simulink library "ESTS_UOD"  (R2024b)
settings: Solver=VariableStepAuto  StartTime=0.0  StopTime=10.0  RelTol=1e-3
libraries: ESTS_UOD_YawRateDeadZone x1, ESTS_UOD_CornrgDir x1, ESTS_UOD_YawRateDifLatRef x1, ESTS_UOD_AgrVSideSlipReDifLatRef x1, ESTS_UOD_FacUnderSteer x1, ESTS_UOD_FacOverSteer x1, VUT_lib x1
settings Model: Creator=blatak  LastModifiedBy=blatak
settings ModelReferenceCC: EnableRefExpFcnMdlSchedulingChecks=on
settings RTWCC: GPUComputeCapability=3.5

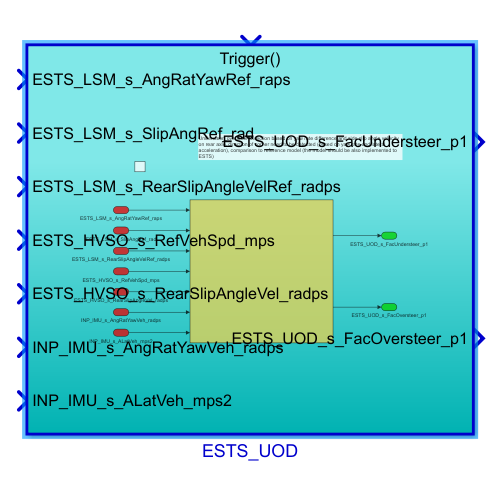
[thumbnail: Simulink's stored preview of the top-level diagram]
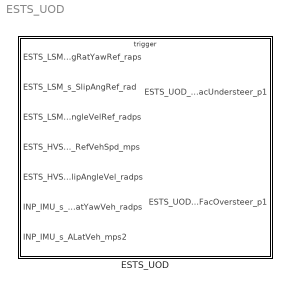
== system ESTS_UOD ==
  ESTS_UOD : Subsystem

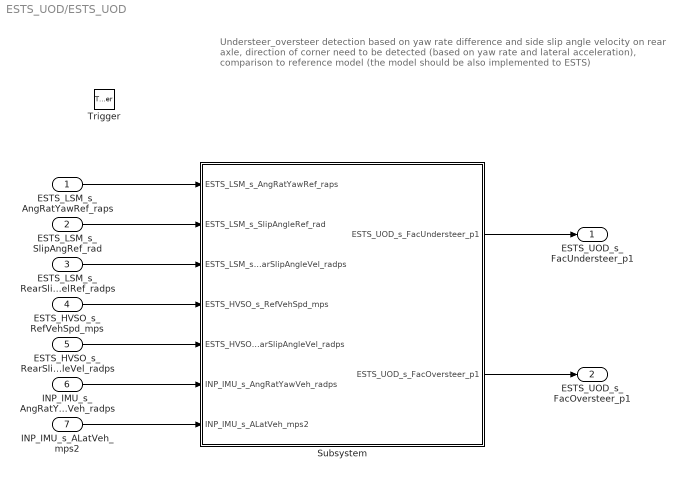
== system ESTS_UOD/ESTS_UOD ==
  note: Understeer_oversteer detection based on yaw rate difference and side slip angle velocity on rear axle, direction of corner need to be detected (based on yaw rate and lateral acceleration), comparison to reference model (the model should be also implemented to ESTS)
  ESTS_LSM_s_AngRatYawRef_raps : Inport
  ESTS_LSM_s_SlipAngRef_rad : Inport  Port=2
  ESTS_LSM_s_RearSlipAngleVelRef_radps : Inport  Port=3
  ESTS_HVSO_s_RefVehSpd_mps : Inport  Port=4
  ESTS_HVSO_s_RearSlipAngleVel_radps : Inport  Port=5
  INP_IMU_s_AngRatYawVeh_radps : Inport  Port=6
  INP_IMU_s_ALatVeh_mps2 : Inport  Port=7
  Trigger : TriggerPort  TriggerType=function-call  VariantControl=(inherit)  PortDimensions=1
  Subsystem : Subsystem
  ESTS_UOD_s_FacUndersteer_p1 : Outport
  ESTS_UOD_s_FacOversteer_p1 : Outport  Port=2
  wires:
  ESTS_LSM_s_RearSlipAngleVelRef_radps/1 -> Subsystem/3(ESTS_LSM_s_RearSlipAngleVel_radps)
  ESTS_HVSO_s_RefVehSpd_mps/1 -> Subsystem/4(ESTS_HVSO_s_RefVehSpd_mps)
  ESTS_HVSO_s_RearSlipAngleVel_radps/1 -> Subsystem/5(ESTS_HVSO_s_RearSlipAngleVel_radps)
  ESTS_LSM_s_SlipAngRef_rad/1 -> Subsystem/2(ESTS_LSM_s_SlipAngleRef_rad)
  ESTS_LSM_s_AngRatYawRef_raps/1 -> Subsystem/1(ESTS_LSM_s_AngRatYawRef_raps)
  Subsystem/2(ESTS_UOD_s_FacOversteer_p1) -> ESTS_UOD_s_FacOversteer_p1/1
  Subsystem/1(ESTS_UOD_s_FacUndersteer_p1) -> ESTS_UOD_s_FacUndersteer_p1/1
  INP_IMU_s_AngRatYawVeh_radps/1 -> Subsystem/6(INP_IMU_s_AngRatYawVeh_radps)
  INP_IMU_s_ALatVeh_mps2/1 -> Subsystem/7(INP_IMU_s_ALatVeh_mps2)

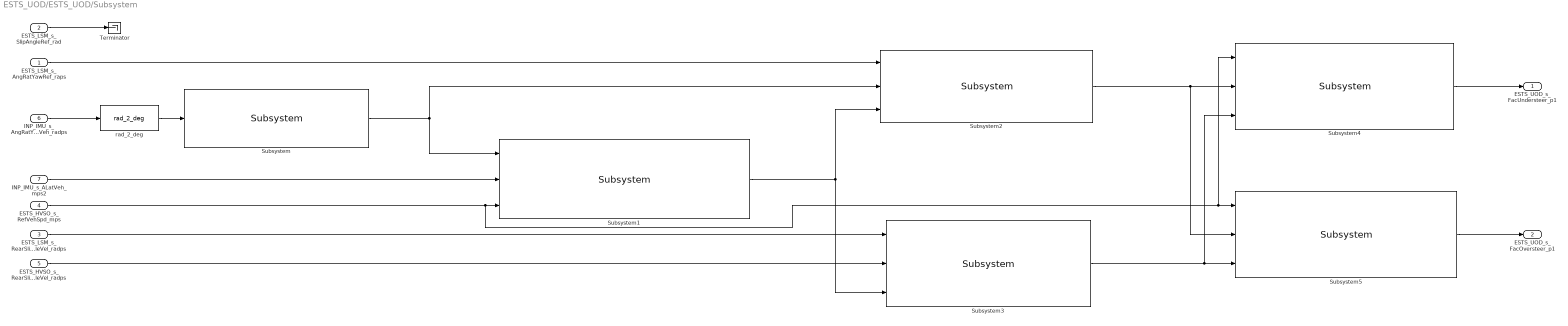
== system ESTS_UOD/ESTS_UOD/Subsystem ==
  ESTS_LSM_s_AngRatYawRef_raps : Inport
  ESTS_LSM_s_SlipAngleRef_rad : Inport  Port=2
  ESTS_LSM_s_RearSlipAngleVel_radps : Inport  Port=3
  ESTS_HVSO_s_RefVehSpd_mps : Inport  Port=4
  ESTS_HVSO_s_RearSlipAngleVel_radps : Inport  Port=5
  INP_IMU_s_AngRatYawVeh_radps : Inport  Port=6
  INP_IMU_s_ALatVeh_mps2 : Inport  Port=7
  Subsystem : ESTS_UOD_YawRateDeadZone/Subsystem  SystemSampleTime=-1  VariantActivationTime=update diagram  AllowFlexibleInterface=on  Latency=0  AutoFrameSizeCalculation=off
  Subsystem1 : ESTS_UOD_CornrgDir/Subsystem  SystemSampleTime=-1  VariantActivationTime=update diagram  AllowFlexibleInterface=on  Latency=0  AutoFrameSizeCalculation=off
  Subsystem2 : ESTS_UOD_YawRateDifLatRef/Subsystem  SystemSampleTime=-1  VariantActivationTime=update diagram  AllowFlexibleInterface=on  Latency=0  AutoFrameSizeCalculation=off
  Subsystem3 : ESTS_UOD_AgrVSideSlipReDifLatRef/Subsystem  SystemSampleTime=-1  VariantActivationTime=update diagram  AllowFlexibleInterface=on  Latency=0  AutoFrameSizeCalculation=off
  Subsystem4 : ESTS_UOD_FacUnderSteer/Subsystem  SystemSampleTime=-1  VariantActivationTime=update diagram  AllowFlexibleInterface=on  Latency=0  AutoFrameSizeCalculation=off
  Subsystem5 : ESTS_UOD_FacOverSteer/Subsystem  SystemSampleTime=-1  VariantActivationTime=update diagram  AllowFlexibleInterface=on  Latency=0  AutoFrameSizeCalculation=off
  Terminator : Terminator
  rad_2_deg : VUT_lib/rad_2_deg  SystemSampleTime=-1  VariantActivationTime=update diagram  AllowFlexibleInterface=on  Latency=0  AutoFrameSizeCalculation=off
  ESTS_UOD_s_FacUndersteer_p1 : Outport
  ESTS_UOD_s_FacOversteer_p1 : Outport  Port=2
  wires:
  INP_IMU_s_AngRatYawVeh_radps/1 -> rad_2_deg/1
  rad_2_deg/1 -> Subsystem/1
  INP_IMU_s_ALatVeh_mps2/1 -> Subsystem1/2
  Subsystem/1 -> Subsystem1/1, Subsystem2/2
  ESTS_LSM_s_RearSlipAngleVel_radps/1 -> Subsystem3/1
  ESTS_LSM_s_SlipAngleRef_rad/1 -> Terminator/1
  ESTS_HVSO_s_RearSlipAngleVel_radps/1 -> Subsystem3/2
  Subsystem1/1 -> Subsystem3/3, Subsystem2/3
  ESTS_LSM_s_AngRatYawRef_raps/1 -> Subsystem2/1
  Subsystem3/1 -> Subsystem4/3, Subsystem5/3
  Subsystem2/1 -> Subsystem5/2, Subsystem4/2
  Subsystem4/1 -> ESTS_UOD_s_FacUndersteer_p1/1
  Subsystem5/1 -> ESTS_UOD_s_FacOversteer_p1/1
  ESTS_HVSO_s_RefVehSpd_mps/1 -> Subsystem4/1, Subsystem5/1, Subsystem1/3
